simulink model "zaibo_ver2"  (R2017b)
settings: Solver=VariableStepAuto  StartTime=0.0  StopTime=0.02  RelTol=1e-3
libraries: powerlib_meascontrol x4
settings Model: Creator=Administrator  LastModifiedBy=zsrx

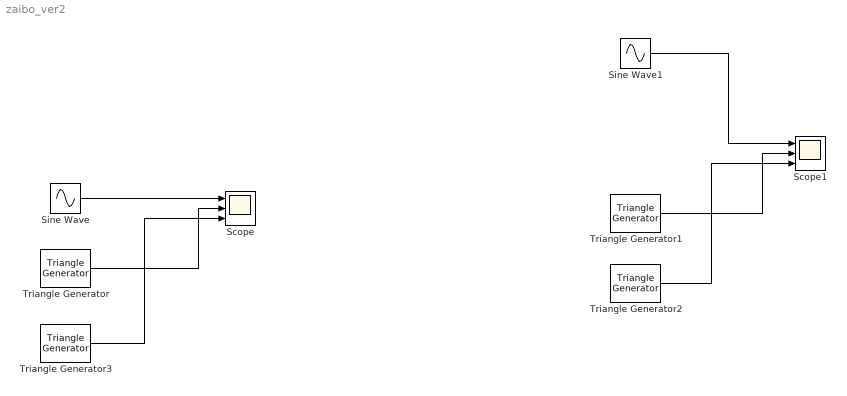
== system zaibo_ver2 ==
  Scope : Scope  NumInputPorts=3
  Scope1 : Scope  NumInputPorts=3
  Sine Wave : Sin  Amplitude=0.9  Frequency=100*pi  SampleTime=0
  Sine Wave1 : Sin  Amplitude=0.9  Frequency=100*pi  SampleTime=0
  Triangle Generator : powerlib_meascontrol/Pulse & Signal Generators/Triangle Generator  Freq=200  Phase=90  Ts=0
  Triangle Generator1 : powerlib_meascontrol/Pulse & Signal Generators/Triangle Generator  Freq=600  Phase=90  Ts=0
  Triangle Generator2 : powerlib_meascontrol/Pulse & Signal Generators/Triangle Generator  Freq=600  Phase=-90  Ts=0
  Triangle Generator3 : powerlib_meascontrol/Pulse & Signal Generators/Triangle Generator  Freq=200  Phase=-90  Ts=0
  wires:
  Sine Wave/1 -> Scope/1
  Sine Wave1/1 -> Scope1/1
  Triangle Generator1/1 -> Scope1/2
  Triangle Generator2/1 -> Scope1/3
  Triangle Generator/1 -> Scope/2
  Triangle Generator3/1 -> Scope/3
